simulink library "saturateWingAngle"  (R2018a)
settings: Solver=VariableStepAuto  StartTime=0.0  StopTime=10.0  RelTol=1e-3
undefined symbols (not defined in the file): plant
libraries: simulink x1
settings Model: Creator=mitch  LastModifiedBy=mitch

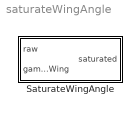
== system saturateWingAngle ==
  SaturateWingAngle : Subsystem

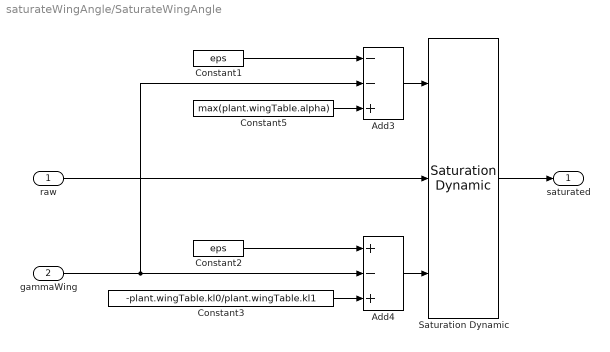
== system saturateWingAngle/SaturateWingAngle ==
  raw : Inport
  gammaWing : Inport  Port=2
  Add3 : Sum  Inputs=--+
  Add4 : Sum  Inputs=+-+
  Constant1 : Constant  Value=eps
  Constant2 : Constant  Value=eps
  Constant3 : Constant  Value=-plant.wingTable.kl0/plant.wingTable.kl1
  Constant5 : Constant  Value=max(plant.wingTable.alpha)
  Saturation Dynamic : simulink/Discontinuities/Saturation Dynamic  OutMin=[]  OutMax=[]  OutDataTypeStr=Inherit: Same as second input  OutDataType=fixdt(1, 16)  OutScaling=2^-10  DoSatur=off
  saturated : Outport
  wires:
  Constant2/1 -> Add4/1
  Constant1/1 -> Add3/1
  Add4/1 -> Saturation Dynamic/3
  Constant3/1 -> Add4/3
  gammaWing/1 -> Add3/2, Add4/2
  Add3/1 -> Saturation Dynamic/1
  Constant5/1 -> Add3/3
  raw/1 -> Saturation Dynamic/2
  Saturation Dynamic/1 -> saturated/1
